simulink model "Simulation"  (R2020a)
settings: Solver=ode4  StartTime=0.0  StopTime=20  FixedStep=0.0001  RelTol=1e-3
libraries: simulink x2
settings Model: Creator=sujay  LastModifiedBy=sujay

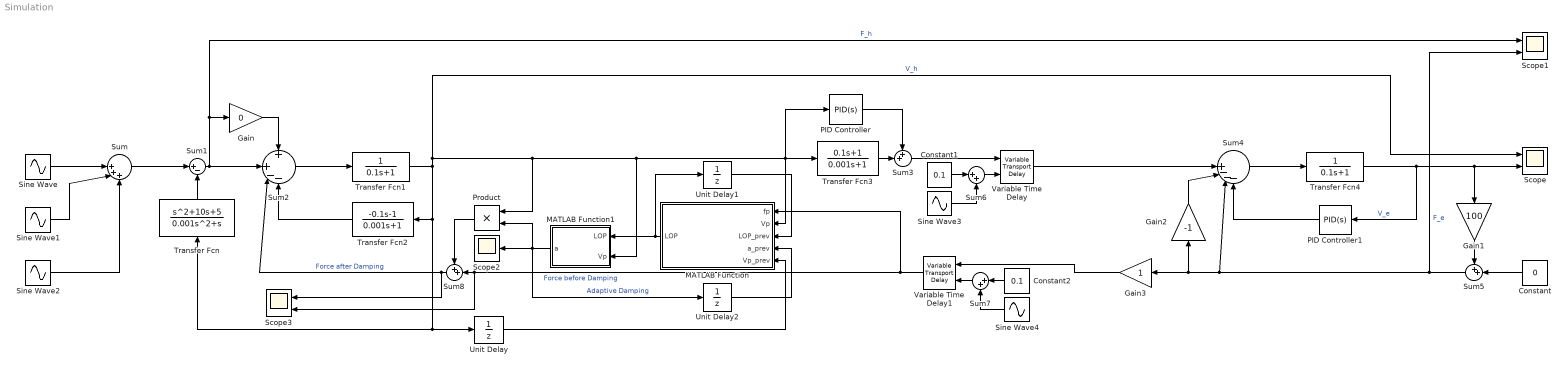
== system Simulation ==
  Constant : Constant  Value=0
  Constant1 : Constant  Value=0.1
  Constant2 : Constant  Value=0.1
  Gain : Gain  Gain=0
  Gain1 : Gain  Gain=100
  Gain2 : Gain  Gain=-1
  Gain3 : Gain
  MATLAB Function : MATLAB Function  TreatAsAtomicUnit=on
  MATLAB Function1 : MATLAB Function  TreatAsAtomicUnit=on
  PID Controller : simulink/Continuous/PID Controller  Controller=PID  Form=Parallel  TimeDomain=Continuous-time  UseExternalTs=off  SampleTime=-1  IntegratorMethod=Forward Euler  FilterMethod=Forward Euler  ControllerParametersSource=internal  P=10  I=0  D=1  UseFilter=on  N=1000  TunerSelectOption=Transfer Function Based (PID Tuner App)  InitialConditionSource=internal  InitialConditionForIntegrator=0  InitialConditionForFilter=0  DifferentiatorICPrevScaledInput=0  ExternalReset=none  TrackingMode=off  Kt=1  LimitOutput=off  UpperSaturationLimit=inf  LowerSaturationLimit=-inf  LinearizeAsGain=on  AntiWindupMode=none  Kb=1  POutMin=[]  POutMax=[]  IOutMin=[]  IOutMax=[]  DOutMin=[]  DOutMax=[]  NOutMin=[]  NOutMax=[]  SumOutMin=[]  SumOutMax=[]  SaturationOutMin=[]  SaturationOutMax=[]  PParamMin=[]  PParamMax=[]  IParamMin=[]  IParamMax=[]  DParamMin=[]  DParamMax=[]  NParamMin=[]  NParamMax=[]  KbParamMin=[]  KbParamMax=[]  KtParamMin=[]  KtParamMax=[]  KbOutMin=[]  KbOutMax=[]  KtOutMin=[]  KtOutMax=[]  IntegratorOutMin=[]  IntegratorOutMax=[]  FilterOutMin=[]  FilterOutMax=[]  SumI1OutMin=[]  SumI1OutMax=[]  SumI2OutMin=[]  SumI2OutMax=[]  SumI3OutMin=[]  SumI3OutMax=[]  SumI4OutMin=[]  SumI4OutMax=[]  SumDOutMin=[]  SumDOutMax=[]  DifferentiatorOutMin=[]  DifferentiatorOutMax=[]  FilterDiffOutCoefMin=[]  FilterDiffOutCoefMax=[]  ReciprocalOutMin=[]  ReciprocalOutMax=[]  SumDenOutMin=[]  SumDenOutMax=[]  SumNumOutMin=[]  SumNumOutMax=[]  DivideOutMin=[]  DivideOutMax=[]  UdiffTsProdOutMin=[]  UdiffTsProdOutMax=[]  NTsProdOutMin=[]  NTsProdOutMax=[]  UintegralTsProdOutMin=[]  UintegralTsProdOutMax=[]  UngainTsProdOutMin=[]  UngainTsProdOutMax=[]  IntegratorContinuousStateAttributes=''  IntegratorStateMustResolveToSignalObject=off  IntegratorRTWStateStorageClass=Auto  FilterContinuousStateAttributes=''  FilterStateMustResolveToSignalObject=off  FilterRTWStateStorageClass=Auto  ParallelPVariant=InternalParameters  IdealPVariant=Disabled  IVariant=InternalParameters  DVariant=InternalParameters  IntegratorVariant=Continuous  SatVariant=Disabled  AWVariant=Passthrough  PCopyVariant=Disabled  TRVariant=Disabled  FdbkBlocksVariant=Forward  IdealPFdbkVariant=Disabled  SatFdbkVariant=Disabled  DerivativeFilterVariant=ContFilter  NVariant=InternalParameters  NCopyVariant=Disabled  FilterICVariant=InternalICsFilter  IntegratorICVariant=InternalICs  ExternalResetVariant=Disabled  TRSumVariant=Passthrough  SumFdbkVariant=Disabled  SumVariant=Sum_PID  TsampFilterVariant=InternalTs  TsampNgainVariant=Passthrough  TsampIntegralVariant=Passthrough
  PID Controller1 : simulink/Continuous/PID Controller  Controller=PID  Form=Parallel  TimeDomain=Continuous-time  UseExternalTs=off  SampleTime=-1  IntegratorMethod=Forward Euler  FilterMethod=Forward Euler  ControllerParametersSource=internal  P=10  I=0  D=1  UseFilter=on  N=1000  TunerSelectOption=Transfer Function Based (PID Tuner App)  InitialConditionSource=internal  InitialConditionForIntegrator=0  InitialConditionForFilter=0  DifferentiatorICPrevScaledInput=0  ExternalReset=none  TrackingMode=off  Kt=1  LimitOutput=off  UpperSaturationLimit=inf  LowerSaturationLimit=-inf  LinearizeAsGain=on  AntiWindupMode=none  Kb=1  POutMin=[]  POutMax=[]  IOutMin=[]  IOutMax=[]  DOutMin=[]  DOutMax=[]  NOutMin=[]  NOutMax=[]  SumOutMin=[]  SumOutMax=[]  SaturationOutMin=[]  SaturationOutMax=[]  PParamMin=[]  PParamMax=[]  IParamMin=[]  IParamMax=[]  DParamMin=[]  DParamMax=[]  NParamMin=[]  NParamMax=[]  KbParamMin=[]  KbParamMax=[]  KtParamMin=[]  KtParamMax=[]  KbOutMin=[]  KbOutMax=[]  KtOutMin=[]  KtOutMax=[]  IntegratorOutMin=[]  IntegratorOutMax=[]  FilterOutMin=[]  FilterOutMax=[]  SumI1OutMin=[]  SumI1OutMax=[]  SumI2OutMin=[]  SumI2OutMax=[]  SumI3OutMin=[]  SumI3OutMax=[]  SumI4OutMin=[]  SumI4OutMax=[]  SumDOutMin=[]  SumDOutMax=[]  DifferentiatorOutMin=[]  DifferentiatorOutMax=[]  FilterDiffOutCoefMin=[]  FilterDiffOutCoefMax=[]  ReciprocalOutMin=[]  ReciprocalOutMax=[]  SumDenOutMin=[]  SumDenOutMax=[]  SumNumOutMin=[]  SumNumOutMax=[]  DivideOutMin=[]  DivideOutMax=[]  UdiffTsProdOutMin=[]  UdiffTsProdOutMax=[]  NTsProdOutMin=[]  NTsProdOutMax=[]  UintegralTsProdOutMin=[]  UintegralTsProdOutMax=[]  UngainTsProdOutMin=[]  UngainTsProdOutMax=[]  IntegratorContinuousStateAttributes=''  IntegratorStateMustResolveToSignalObject=off  IntegratorRTWStateStorageClass=Auto  FilterContinuousStateAttributes=''  FilterStateMustResolveToSignalObject=off  FilterRTWStateStorageClass=Auto  ParallelPVariant=InternalParameters  IdealPVariant=Disabled  IVariant=InternalParameters  DVariant=InternalParameters  IntegratorVariant=Continuous  SatVariant=Disabled  AWVariant=Passthrough  PCopyVariant=Disabled  TRVariant=Disabled  FdbkBlocksVariant=Forward  IdealPFdbkVariant=Disabled  SatFdbkVariant=Disabled  DerivativeFilterVariant=ContFilter  NVariant=InternalParameters  NCopyVariant=Disabled  FilterICVariant=InternalICsFilter  IntegratorICVariant=InternalICs  ExternalResetVariant=Disabled  TRSumVariant=Passthrough  SumFdbkVariant=Disabled  SumVariant=Sum_PID  TsampFilterVariant=InternalTs  TsampNgainVariant=Passthrough  TsampIntegralVariant=Passthrough
  Product : Product
  Scope : Scope  NumInputPorts=2
  Scope1 : Scope  NumInputPorts=2
  Scope2 : Scope
  Scope3 : Scope  NumInputPorts=2
  Sine Wave : Sin  Frequency=2  SampleTime=0
  Sine Wave1 : Sin  Amplitude=0.25  Frequency=6  Phase=pi/2  SampleTime=0
  Sine Wave2 : Sin  Amplitude=0.1  Frequency=18  SampleTime=0
  Sine Wave3 : Sin  Amplitude=0.02  Frequency=12  SampleTime=0
  Sine Wave4 : Sin  Amplitude=0.02  Frequency=12  SampleTime=0
  Sum : Sum  Inputs=||+++
  Sum1 : Sum  Inputs=|+-
  Sum2 : Sum  Inputs=+|+--
  Sum3 : Sum  Inputs=++|
  Sum4 : Sum  Inputs=|||+---
  Sum5 : Sum  Inputs=++|
  Sum6 : Sum  Inputs=|++
  Sum7 : Sum  Inputs=|++
  Sum8 : Sum  Inputs=++|
  Transfer Fcn : TransferFcn  Numerator=[1,10,5]  Denominator=[0.001,1,0]
  Transfer Fcn1 : TransferFcn  Denominator=[0.1,1]
  Transfer Fcn2 : TransferFcn  Numerator=[-0.1,-1]  Denominator=[0.001,1]
  Transfer Fcn3 : TransferFcn  Numerator=[0.1,1]  Denominator=[0.001,1]
  Transfer Fcn4 : TransferFcn  Denominator=[0.1,1]
  Unit Delay : UnitDelay  SampleTime=0.0001  HasFrameUpgradeWarning=on
  Unit Delay1 : UnitDelay  SampleTime=0.0001  HasFrameUpgradeWarning=on
  Unit Delay2 : UnitDelay  SampleTime=0.0001  HasFrameUpgradeWarning=on
  Variable Time Delay : VariableTransportDelay  MaximumDelay=10  MaximumPoints=2048
  Variable Time Delay1 : VariableTransportDelay  MaximumDelay=10  MaximumPoints=2048
  wires:
  Sine Wave/1 -> Sum/1
  Sine Wave1/1 -> Sum/2
  Sine Wave2/1 -> Sum/3
  Sum/1 -> Sum1/1
  Transfer Fcn/1 -> Sum1/2
  Sum1/1 -> Gain/1, Scope1/1, Sum2/2  "F_h"
  Gain/1 -> Sum2/1
  Sum2/1 -> Transfer Fcn1/1
  Transfer Fcn2/1 -> Sum2/4
  PID Controller/1 -> Sum3/1
  Transfer Fcn3/1 -> Sum3/2
  Sum4/1 -> Transfer Fcn4/1
  Transfer Fcn4/1 -> Scope/2, Gain1/1, PID Controller1/1  "V_e"
  PID Controller1/1 -> Sum4/4
  Constant/1 -> Sum5/2
  Gain1/1 -> Sum5/1
  Sum5/1 -> Scope1/2, Gain3/1, Gain2/1, Sum4/3  "F_e"
  Gain2/1 -> Sum4/2
  Sum6/1 -> Variable Time Delay/2
  Constant1/1 -> Sum6/1
  Sine Wave3/1 -> Sum6/2
  Sum7/1 -> Variable Time Delay1/2
  Constant2/1 -> Sum7/1
  Sine Wave4/1 -> Sum7/2
  Variable Time Delay/1 -> Sum4/1
  Gain3/1 -> Variable Time Delay1/1
  MATLAB Function/1(LOP) -> MATLAB Function1/1(LOP), Unit Delay1/1
  Sum8/1 -> Scope3/1, Sum2/3  "Force after Damping"
  Product/1 -> Sum8/1
  Sum3/1 -> Variable Time Delay/1
  Transfer Fcn1/1 -> Product/1, MATLAB Function1/2(Vp), PID Controller/1, Transfer Fcn3/1, MATLAB Function/2(Vp), Scope/1, Transfer Fcn2/1, Transfer Fcn/1, Unit Delay/1  "V_h"
  Unit Delay1/1 -> MATLAB Function/3(LOP_prev)
  Variable Time Delay1/1 -> MATLAB Function/1(fp), Scope3/2, Sum8/2  "Force before Damping"
  MATLAB Function1/1(a) -> Scope2/1, Product/2, Unit Delay2/1  "Adaptive Damping"
  Unit Delay2/1 -> MATLAB Function/4(a_prev)
  Unit Delay/1 -> MATLAB Function/5(Vp_prev)

== matlab function Simulation/MATLAB Function1 ==
  data: LOP input; a output; Vp input
function a = Stabilizer(LOP,Vp)

dt = 0.0001;

if LOP < 0
    if Vp ~= 0
        a = -LOP/(Vp*Vp*dt);
    else
        a = 0; 
    end
else
    a = 0;
end

end

== matlab function Simulation/MATLAB Function ==
  data: fp input; LOP output; Vp input; LOP_prev input; a_prev input; Vp_prev input
function LOP = PO(fp,Vp,LOP_prev,a_prev,Vp_prev)

f = 0.99;
dt = 0.0001;

P_L = ( 3 - 0.5 )*Vp*Vp + fp*Vp;
LOP = f*LOP_prev + (P_L + f*a_prev*Vp_prev*Vp_prev)*dt;

end
